simulink model "aMPC_for_embedded"  (R2019a)
settings: Solver=ode1  StartTime=0.0  StopTime=20  FixedStep=0.01  RelTol=1e-3  EnableMultiTasking=on
libraries: mpclib x1, simulink x1
settings Model: Creator=alexh  LastModifiedBy=alexh
settings SolverCC: PositivePriorityOrder=on  AutoInsertRateTranBlk=on
settings OptimizationCC: EnhancedBackFolding=on  PassReuseOutputArgsAs=Individual arguments  MaxStackSize=64  OptimizeBlockOrder=speed  DifferentSizesBufferReuse=on  OptimizationCustomize=off
settings DebuggingCC: ParameterTunabilityLossMsg=error
settings HardwareCC: ProdBitPerPointer=32  ProdBitPerSizeT=32  ProdBitPerPtrDiffT=32  ProdLargestAtomicInteger=Long  ProdLargestAtomicFloat=Double  ProdWordSize=32  ProdLongLongMode=on  ProdHWDeviceType=ARM Compatible->ARM Cortex  UseEmbeddedCoderFeatures=off
settings SFSimCC: MATLABDynamicMemAlloc=off
settings RTWCC: SystemTargetFile=ert.tlc  HardwareBoard=Raspberry Pi  TLCOptions="-aInlineSetEventsForThisBaseRateFcn=TLC_FALSE -aSuppressMultiTaskScheduler=TLC_FALSE  -aRateBasedStepFcn=0"  TemplateMakefile=ert_default_tmf  GenerateReport=on  Toolchain=GNU GCC Raspberry Pi  BuildConfiguration=Debug  IncludeHyperlinkInReport=on  LaunchReport=on  TargetLang=C++  GenerateTraceInfo=on  GenerateTraceReport=on  GenerateTraceReportSl=on  GenerateTraceReportSf=on  GenerateTraceReportEml=on
settings CodeAppCC: ForceParamTrailComments=on  IgnoreCustomStorageClasses=off  OperatorAnnotations=on  SimulinkDataObjDesc=on  SFDataObjDesc=on  InsertBlockDesc=on
settings ERTTargetCC: TargetLangStandard=C++03 (ISO)  MultiInstanceERTCode=on  CodeInterfacePackaging=C++ class  SupportNonInlinedSFcns=on  SupportVariableSizeSignals=on

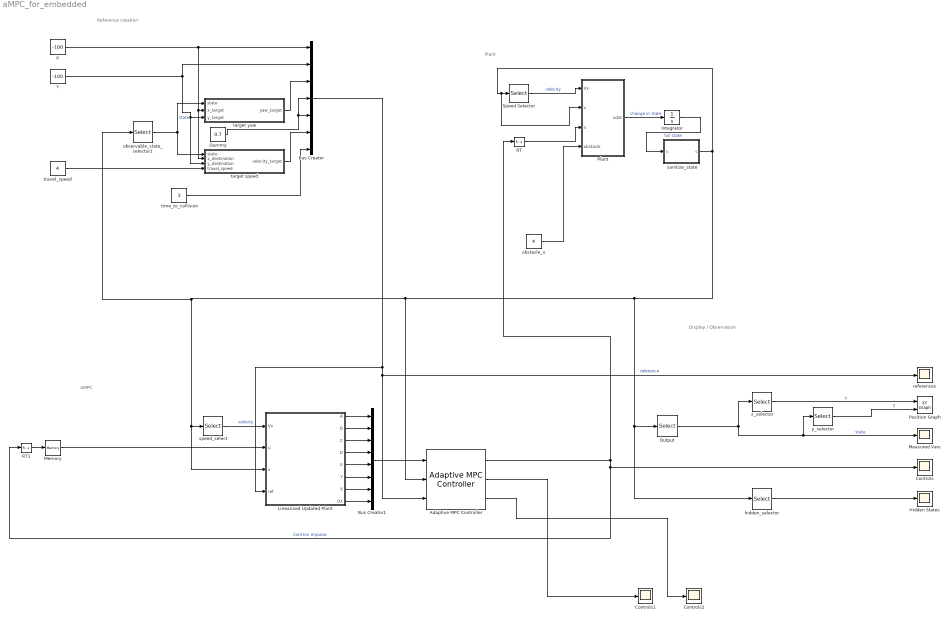
== system aMPC_for_embedded ==
  note: aMPC
  note: Plant
  note: Reference creation
  note: Display / Observation
  Adaptive MPC Controller : mpclib/Adaptive MPC Controller  SCDEnableBlockLinearizationSpecification=on  mpcobj=cv_mpc  enable_value=0  updateMPCinCallerWorkspace=on  md_inport=off  mv_inport=off  uref_inport=off  return_cost=on  return_mvseq=off  return_qpstatus=off  return_xseq=off  return_state=on  return_ovseq=off  state_inport=off  isltv_plant=off  umin_inport=off  umax_inport=off  ymin_inport=off  ymax_inport=off  cc_inport=off  ywt_inport=off  uwt_inport=off  duwt_inport=off  rhoeps_inport=off  pm_inport=off  MaximumP=10  HorizonChoice=FixedHorizon  BlockDataType=double  SampleTimeInherited=off  switch_inport=off
      settings: SourceProductName=MATLAB Runtime - Model Predictive Control Toolbox Addin  SourceProductBaseCode=Missing
  Bus Creator : BusCreator  Inputs=7
  Bus Creator1 : BusCreator  Inputs=8
  Controls : Scope
  Controls1 : Scope
  Controls2 : Scope
  Dummy : Constant  Value=0.7
  Hidden States : Scope
  Integrator : Integrator
  Linearized Updated Plant : MATLAB Function  TreatAsAtomicUnit=on
  Measured Vars : Scope
  Memory : Memory
  Output : Selector  InputPortWidth=7  IndexOptions=Index vector (dialog)  Indices=[1, 2, 3, 6, 7]  OutputSizes=1
  "Plant " : MATLAB Function  TreatAsAtomicUnit=on
  Position Graph : simulink/Sinks/XY Graph  xmin=-15  xmax=15  ymin=-15  ymax=15  st=-1
  RT : RateTransition  OutPortSampleTime=0.01
  RT1 : RateTransition  OutPortSampleTime=0.01
  Speed Selector : Selector  InputPortWidth=7  IndexOptions=Index vector (dialog)  Indices=[6]  OutputSizes=1
  X : Constant  Value=-100
  Y : Constant  Value=-100
  hidden_selector : Selector  InputPortWidth=7  IndexOptions=Index vector (dialog)  Indices=[4, 5]  OutputSizes=1
  observable_state_selector1 : Selector  InputPortWidth=7  IndexOptions=Index vector (dialog)  Indices=[1, 2, 3, 6]  OutputSizes=1
  obstacle_x : Constant  Value=4
  references : Scope
  sanitize_state : MATLAB Function  TreatAsAtomicUnit=on
  speed_select : Selector  InputPortWidth=7  IndexOptions=Index vector (dialog)  Indices=[6]  OutputSizes=1
  target speed : MATLAB Function  TreatAsAtomicUnit=on
  target yaw : MATLAB Function  TreatAsAtomicUnit=on
  time_to_collision : Constant  Value=3
  travel_speed : Constant  Value=4
  x_selector : Selector  InputPortWidth=5  IndexOptions=Index vector (dialog)  Indices=[1]  OutputSizes=1
  y_selector : Selector  InputPortWidth=5  IndexOptions=Index vector (dialog)  Indices=[2]  OutputSizes=1
  wires:
  "Plant "/1(xdot) -> Integrator/1  "change in state"
  target speed/1(velocity_target) -> Bus Creator/6
  target yaw/1(yaw_target) -> Bus Creator/3
  Linearized Updated Plant/5(U) -> Bus Creator1/5
  Linearized Updated Plant/4(D) -> Bus Creator1/4
  Output/1 -> x_selector/1, Measured Vars/1, y_selector/1  "state"
  Linearized Updated Plant/3(C) -> Bus Creator1/3
  Linearized Updated Plant/1(A) -> Bus Creator1/1
  Bus Creator1/1 -> Adaptive MPC Controller/1
  Linearized Updated Plant/2(B) -> Bus Creator1/2
  Linearized Updated Plant/8(DX) -> Bus Creator1/8
  Linearized Updated Plant/7(X) -> Bus Creator1/7
  Adaptive MPC Controller/1 -> RT/1, RT1/1, Controls/1  "Contron Impulse"
  Memory/1 -> Linearized Updated Plant/2(u)
  x_selector/1 -> Position Graph/1  "x"
  Bus Creator/1 -> Adaptive MPC Controller/3, references/1, Linearized Updated Plant/4(ref)  "reference"
  y_selector/1 -> Position Graph/2  "y"
  hidden_selector/1 -> Hidden States/1
  travel_speed/1 -> target speed/4(travel_speed)
  Linearized Updated Plant/6(Y) -> Bus Creator1/6
  Integrator/1 -> sanitize_state/1("s ")  "full state"
  Y/1 -> target speed/3(y_destination), target yaw/3(y_target), Bus Creator/2
  Speed Selector/1 -> "Plant "/1(Vx)  "velocity"
  X/1 -> target speed/2(x_destination), target yaw/2(x_target), Bus Creator/1
  RT/1 -> "Plant "/3(u)
  RT1/1 -> Memory/1
  speed_select/1 -> Linearized Updated Plant/1(Vx)  "velocity"
  observable_state_selector1/1 -> target speed/1(state), target yaw/1(state)  "state"
  Dummy/1 -> Bus Creator/5, Bus Creator/4
  obstacle_x/1 -> "Plant "/4(obstacle)
  time_to_collision/1 -> Bus Creator/7
  sanitize_state/1(s) -> "Plant "/2(x), Speed Selector/1, observable_state_selector1/1, Linearized Updated Plant/3(x), speed_select/1, Adaptive MPC Controller/2, hidden_selector/1, Output/1
  Adaptive MPC Controller/2 -> Controls1/1
  Adaptive MPC Controller/3 -> Controls2/1

== matlab function aMPC_for_embedded/Linearized Updated Plant ==
  data: Vx input; u input; A output; x input; B output; C output; D output; U output; Y output; X output; DX output; ref input
function [A,B,C,D,U,Y,X,DX] = fcn(Vx,u,x, ref)

m = 20;     % Mass
lf = 2;   % Distance mass center/front wheel
lr = 2;   % Distance mass center/rear wheel
cf = 3000;   % Cornering Stiffness front
cr = 3000;   % Cornering Stiffness rear
iz = 300;   % Yaw Moment of Innertia?
Ts = 0.1;

if (Vx<0.1)
       Vx = 0.1;
end

% Continuous-time model
Ac = [0, 0, -Vx, 0, -1, 1, 0;     % TODO: Gedanke - Hier kann ich y anders brerechnen wenn y als offset zur mitte definiert wird; abzüglich yaw rate
       0, 0, Vx, 0, 1, 0, 0;
       0, 0, 0, 0, 0, 0, 0;
       0, 0, 0, -(cr*lr^2+cf*lf^2)/iz/Vx, -(cr*lr-cf*lf)/iz, 0, 0;
       0, 0, 0, 1-(cr*lr-cf*lf)/m/Vx^2, -(cf+cr)/m/Vx, 0, 0;
       0, 0, 0, 0, 0, -.1, 0;
       0, 0, 0, 0, 0, -1, 0];
   
Bc = [0, 0, 0, cf*lf/iz, -cf/m/Vx, 0, 0;
        0, 0, 0, 0, 0, 1, 0;
        0, 0, 0, 0, 0, -2, 0]';
 
 % Position, Yaw, Speed
 Cc = [1, 0, 0, 0, 0, 0, 0;
     0, 1, 0, 0, 0, 0, 0;
     0, 0, 1, 0, 0, 0, 0;
     0, 0, 0, 1, 0, 0, 0;
     0, 0, 0, 0, 1, 0, 0;
     0, 0, 0, 0, 0, 1, 0;
     0, 0, 0, 0, 0, 0, 1];
    
 Dc = zeros(7, 3);

% Generate discrete-time model
nx = size(Ac,1);
nu = size(Bc,2);
M = expm([[Ac Bc]*Ts; zeros(nu,nx+nu)]);
A = M(1:nx,1:nx);
B = M(1:nx,nx+1:nx+nu);
C = Cc;
D = Dc;

% Nominal conditions for discrete-time plant
X = x';
U = u';
Y = (C*x + D*u)';
DX = (A*x+B*u-x)';      % did this fix, might be wrong

== matlab function aMPC_for_embedded/Plant  ==
  data: Vx input; x input; u input; xdot output; obstacle input
function xdot = fcn(Vx,x,u, obstacle)

if (Vx<1)
    Vx=1;
end

m = 30;     % Mass
lf = 0.7;   % Distance mass center/front wheel
lr = 0.3;   % Distance mass center/rear wheel
cf = 3000;   % Cornering Stiffness front
cr = 3000;   % Cornering Stiffness rear
iz = 100;   % Yaw Moment of Innertia?

sin_yaw = sin(x(3));
cos_yaw = cos(x(3));


% Continuous-time model
% Continuous-time model
Ac = [0, 0, 0, 0, 0, cos_yaw, 0;
       0, 0, 0, 0, 0, sin_yaw, 0;
       0, 0, 0, 1, 0, 0, 0;
       0, 0, 0, -(cr*lr^2+cf*lf^2)/iz/Vx, -(cr*lr-cf*lf)/iz, 0, 0;
       0, 0, 0, 1-(cr*lr-cf*lf)/m/Vx^2, -(cf+cr)/m/Vx, 0, 0;
       0, 0, 0, 0, 0, -.1, 0;
       0, 0, 0, 0, 0, -1, 0];

   
 Bc = [0, 0, 0, cf*lf/iz, -cf/m/Vx, 0, 0;
        0, 0, 0, 0, 0, 1, 0;
        0, 0, 0, 0, 0, -2, 0]';

xdot = Ac*x + Bc*u;

% Make vehicle stop if obstacle is close
if (obstacle-x) < 1
    xdot(7) = 0;
end

== matlab function aMPC_for_embedded/target yaw ==
  data: state input; yaw_target output; x_target input; y_target input
function yaw_target = fcn(state, x_target, y_target)

% Rearange data
x = state(1);
y = state(2);
yaw = state(3);

% Calculate target yaw
yaw_target = atan2(y_target-y, x_target-x);

% Adjust so we actually take shortest doff
yaw_diff = abs(yaw - yaw_target);

if yaw_diff < pi
    if yaw_target < 0 && yaw > 0
        yaw_target = yaw_target + 2*pi;
    end
    if yaw_target > 0 && yaw < 0
        yaw_target = yaw_target - 2*pi;
    end    
end

== matlab function aMPC_for_embedded/target speed ==
  data: state input; velocity_target output; x_destination input; y_destination input; travel_speed input
function velocity_target = fcn(state, x_destination, y_destination, travel_speed)

% Rearange data
position = [state(1) state(2)];
position_target = [x_destination, y_destination];

% Calculate delta position
delta_position = position - position_target;

distance_to_travel = norm(delta_position);

velocity_target = min(travel_speed, distance_to_travel/2);

== matlab function aMPC_for_embedded/sanitize_state ==
  data: s input; s output
function s = fcn(s)

if (s(3)>pi)
    %s(3) = s(3) - 2*pi;
end
if (s(3)<-pi)
    %s(3) = s(3) + 2*pi;
end
